simulink model "LinearAirframe"  (R2025a)
settings: Solver=VariableStepAuto  StartTime=0.0  StopTime=10.0  FixedStep=0.03  RelTol=1e-3
undefined symbols (not defined in the file): b, d_t, g, l, m
settings Model: Creator=tobia  LastModifiedBy=dma

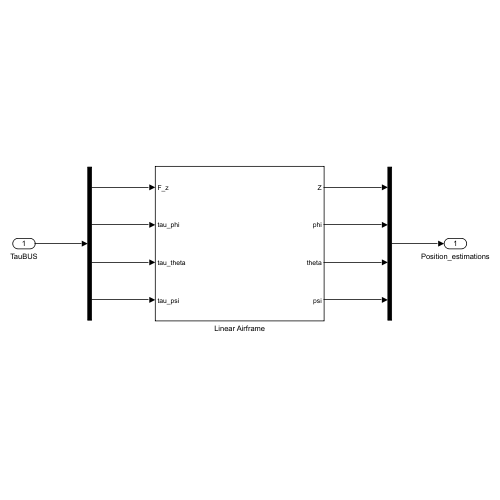
[thumbnail: Simulink's stored preview of the top-level diagram]
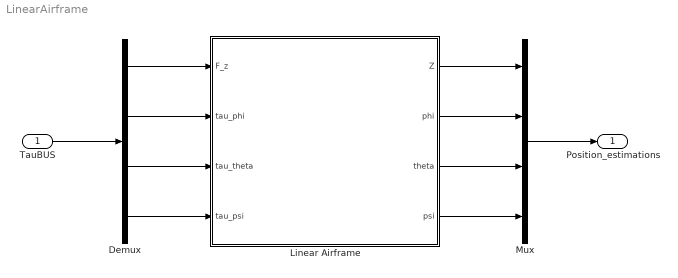
== system LinearAirframe ==
  TauBUS : Inport
  Demux : Demux
  Linear Airframe : Subsystem
  Mux : Mux
  Position_estimations : Outport
  wires:
  Demux/1 -> Linear Airframe/1(F_z)
  Linear Airframe/1(Z) -> Mux/1
  Linear Airframe/2(phi) -> Mux/2
  Linear Airframe/3(theta) -> Mux/3
  Linear Airframe/4(psi) -> Mux/4
  Mux/1 -> Position_estimations/1
  TauBUS/1 -> Demux/1
  Demux/2 -> Linear Airframe/2(tau_phi)
  Demux/3 -> Linear Airframe/3(tau_theta)
  Demux/4 -> Linear Airframe/4(tau_psi)

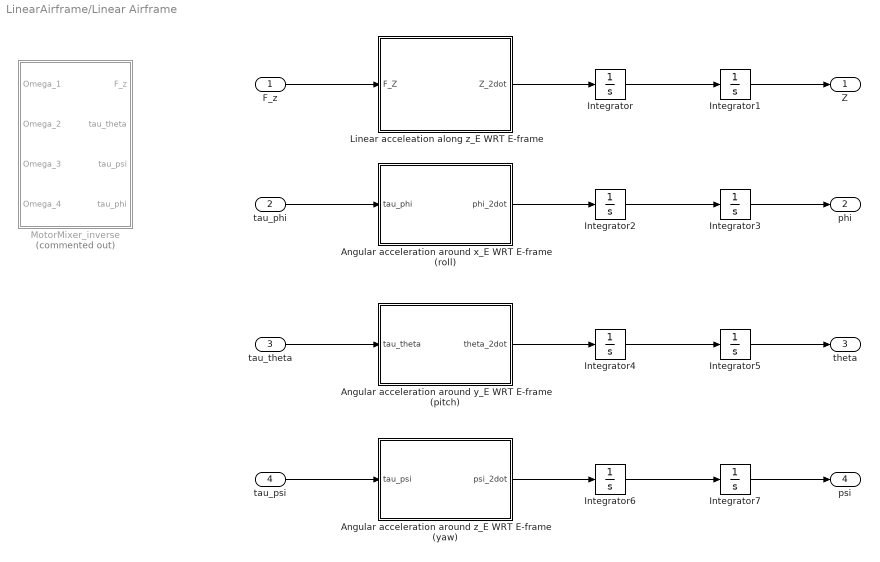
== system LinearAirframe/Linear Airframe ==
  F_z : Inport
  tau_phi : Inport  Port=2
  tau_theta : Inport  Port=3
  tau_psi : Inport  Port=4
  Angular acceleration around x_E WRT E-frame (roll) : MATLAB Function  TreatAsAtomicUnit=on
  Angular acceleration around y_E WRT E-frame (pitch) : MATLAB Function  TreatAsAtomicUnit=on
  Angular acceleration around z_E WRT E-frame (yaw) : MATLAB Function  TreatAsAtomicUnit=on
  Integrator{,1..7} (8 alike) : Integrator
  Linear acceleation along z_E WRT E-frame : MATLAB Function  TreatAsAtomicUnit=on
  MotorMixer_inverse : Subsystem  Commented=on
  Z : Outport
  phi : Outport  Port=2
  theta : Outport  Port=3
  psi : Outport  Port=4
  wires:
  Integrator/1 -> Integrator1/1
  Angular acceleration around z_E WRT E-frame (yaw)/1(psi_2dot) -> Integrator6/1
  Integrator7/1 -> psi/1
  F_z/1 -> Linear acceleation along z_E WRT E-frame/1(F_Z)
  tau_psi/1 -> Angular acceleration around z_E WRT E-frame (yaw)/1(tau_psi)
  Integrator3/1 -> phi/1
  Linear acceleation along z_E WRT E-frame/1(Z_2dot) -> Integrator/1
  tau_phi/1 -> Angular acceleration around x_E WRT E-frame (roll)/1(tau_phi)
  Integrator6/1 -> Integrator7/1
  Integrator1/1 -> Z/1
  Integrator4/1 -> Integrator5/1
  Integrator2/1 -> Integrator3/1
  Angular acceleration around x_E WRT E-frame (roll)/1(phi_2dot) -> Integrator2/1
  Angular acceleration around y_E WRT E-frame (pitch)/1(theta_2dot) -> Integrator4/1
  Integrator5/1 -> theta/1
  tau_theta/1 -> Angular acceleration around y_E WRT E-frame (pitch)/1(tau_theta)

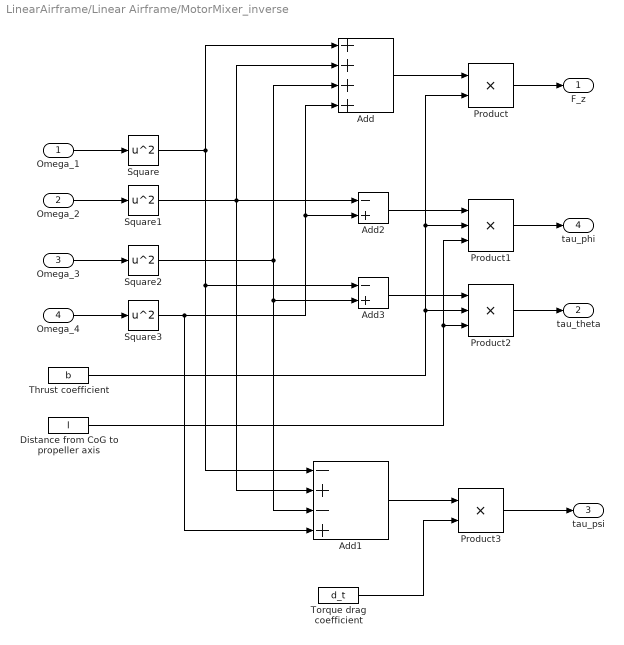
== system LinearAirframe/Linear Airframe/MotorMixer_inverse ==
  Omega_1 : Inport
  Omega_2 : Inport  Port=2
  Omega_3 : Inport  Port=3
  Omega_4 : Inport  Port=4
  Add : Sum  Inputs=++++
  Add1 : Sum  Inputs=-+-+
  Add2 : Sum  Inputs=-+
  Add3 : Sum  Inputs=-+
  Distance from CoG to propeller axis : Constant  Value=l
  Product : Product
  Product1 : Product  Inputs=3
  Product2 : Product  Inputs=3
  Product3 : Product
  Square{,1..3} (4 alike) : Math  Operator=square
  Thrust coefficient : Constant  Value=b
  Torque drag coefficient : Constant  Value=d_t
  F_z : Outport
  tau_theta : Outport  Port=2
  tau_psi : Outport  Port=3
  tau_phi : Outport  Port=4
  wires:
  Omega_1/1 -> Square/1
  Omega_2/1 -> Square1/1
  Omega_3/1 -> Square2/1
  Omega_4/1 -> Square3/1
  Square3/1 -> Add1/4, Add/4, Add2/2
  Square2/1 -> Add/3, Add1/3, Add3/2
  Square1/1 -> Add1/2, Add2/1, Add/2
  Square/1 -> Add1/1, Add3/1, Add/1
  Add/1 -> Product/1
  Thrust coefficient/1 -> Product2/2, Product1/2, Product/2
  Distance from CoG to propeller axis/1 -> Product1/3, Product2/3
  Torque drag coefficient/1 -> Product3/2
  Add2/1 -> Product1/1
  Add3/1 -> Product2/1
  Add1/1 -> Product3/1
  Product3/1 -> tau_psi/1
  Product/1 -> F_z/1
  Product1/1 -> tau_phi/1
  Product2/1 -> tau_theta/1

== matlab function LinearAirframe/Linear Airframe/Angular acceleration around x_E WRT E-frame (roll) ==
  data: tau_phi input; phi_2dot output; I_XX parameter
function phi_2dot = fcn(tau_phi, I_XX)

phi_2dot = tau_phi/I_XX;

== matlab function LinearAirframe/Linear Airframe/Linear acceleation along z_E WRT E-frame ==
  data: F_Z input; Z_2dot output; m parameter; g parameter
function Z_2dot = fcn(F_Z, m, g) 

Z_2dot = -g+F_Z/m;

%g = graviational constant
%m = mass

== matlab function LinearAirframe/Linear Airframe/Angular acceleration around y_E WRT E-frame (pitch) ==
  data: tau_theta input; theta_2dot output; I_YY parameter
function theta_2dot = fcn(tau_theta, I_YY)

theta_2dot = tau_theta/I_YY;

== matlab function LinearAirframe/Linear Airframe/Angular acceleration around z_E WRT E-frame (yaw) ==
  data: tau_psi input; psi_2dot output; I_ZZ parameter
function psi_2dot = fcn(tau_psi, I_ZZ)

psi_2dot = tau_psi/I_ZZ;
